simulink library "WBToolbox2Library_repository"  (R2017a)
settings: Solver=ode45  StartTime=0.0  StopTime=10.0  RelTol=1e-3  EnableMultiTasking=on
undefined symbols (not defined in the file): WBT_modelName, WBT_robotName, WBT_wbiFilename, WBT_wbiList
libraries: simulink x1
(part 2 of 2)

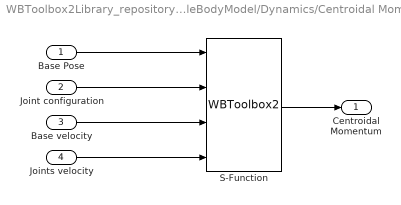
== system WBToolbox2Library_repository/wholeBodyModel/Dynamics/Centroidal Momentum ==
  Base Pose : Inport
  Joint configuration : Inport  Port=2
  Base velocity : Inport  Port=3
  Joints velocity : Inport  Port=4
  S-Function : S-Function  FunctionName=WBToolbox2  Parameters='CentroidalMomentum',robotName,localName,wbiFile,wbiList  SFunctionDeploymentMode=off  EnableBusSupport=off
  Centroidal Momentum : Outport
  wires:
  S-Function/1 -> Centroidal Momentum/1
  Base Pose/1 -> S-Function/1
  Joint configuration/1 -> S-Function/2
  Base velocity/1 -> S-Function/3
  Joints velocity/1 -> S-Function/4

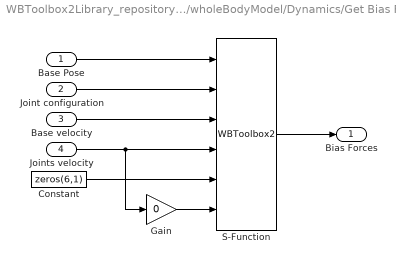
== system WBToolbox2Library_repository/wholeBodyModel/Dynamics/Get Bias Forces ==
  Base Pose : Inport
  Joint configuration : Inport  Port=2
  Base velocity : Inport  Port=3
  Joints velocity : Inport  Port=4
  Constant : Constant  Value=zeros(6,1)
  Gain : Gain  Gain=0
  S-Function : S-Function  FunctionName=WBToolbox2  Parameters='InverseDynamics',robotName,localName,wbiFile,wbiList,explicitGravity  SFunctionDeploymentMode=off  EnableBusSupport=off
  Bias Forces : Outport
  wires:
  S-Function/1 -> Bias Forces/1
  Base Pose/1 -> S-Function/1
  Joint configuration/1 -> S-Function/2
  Base velocity/1 -> S-Function/3
  Joints velocity/1 -> Gain/1, S-Function/4
  Constant/1 -> S-Function/5
  Gain/1 -> S-Function/6

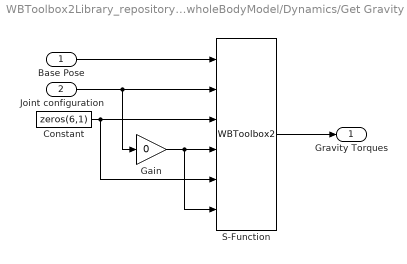
== system WBToolbox2Library_repository/wholeBodyModel/Dynamics/Get Gravity Forces ==
  Base Pose : Inport
  Joint configuration : Inport  Port=2
  Constant : Constant  Value=zeros(6,1)
  Gain : Gain  Gain=0
  S-Function : S-Function  FunctionName=WBToolbox2  Parameters='InverseDynamics',robotName,localName,wbiFile,wbiList,explicitGravity  SFunctionDeploymentMode=off  EnableBusSupport=off
  Gravity Torques : Outport
  wires:
  S-Function/1 -> Gravity Torques/1
  Base Pose/1 -> S-Function/1
  Joint configuration/1 -> Gain/1, S-Function/2
  Constant/1 -> S-Function/5, S-Function/3
  Gain/1 -> S-Function/6, S-Function/4

== system WBToolbox2Library_repository/wholeBodyModel/Dynamics/Mass Matrix ==
  Base Pose : Inport
  Joint configuration : Inport  Port=2
  S-Function : S-Function  FunctionName=WBToolbox2  Parameters='MassMatrix',robotName,localName,wbiFile,wbiList  SFunctionDeploymentMode=off  EnableBusSupport=off
  Mass Matrix : Outport
  wires:
  S-Function/1 -> Mass Matrix/1
  Base Pose/1 -> S-Function/1
  Joint configuration/1 -> S-Function/2

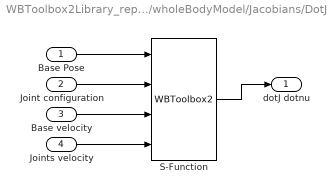
== system WBToolbox2Library_repository/wholeBodyModel/Jacobians/DotJ Nu ==
  Base Pose : Inport
  Joint configuration : Inport  Port=2
  Base velocity : Inport  Port=3
  Joints velocity : Inport  Port=4
  S-Function : S-Function  FunctionName=WBToolbox2  Parameters='DotJNu',robotName,localName,wbiFile,wbiList,frameName  SFunctionDeploymentMode=off  EnableBusSupport=off
  dotJ dotnu : Outport
  wires:
  Joint configuration/1 -> S-Function/2
  Base Pose/1 -> S-Function/1
  S-Function/1 -> dotJ dotnu/1
  Base velocity/1 -> S-Function/3
  Joints velocity/1 -> S-Function/4

== system WBToolbox2Library_repository/wholeBodyModel/Jacobians/Jacobian ==
  Base Pose : Inport
  Joint configuration : Inport  Port=2
  S-Function : S-Function  FunctionName=WBToolbox2  Parameters='Jacobian',robotName,localName,wbiFile,wbiList,frameName  SFunctionDeploymentMode=off  EnableBusSupport=off
  Forward Kinematics : Outport
  wires:
  S-Function/1 -> Forward Kinematics/1
  Base Pose/1 -> S-Function/1
  Joint configuration/1 -> S-Function/2

== system WBToolbox2Library_repository/wholeBodyModel/Kinematics/Forward Kinematics ==
  Base Pose : Inport
  Joint configuration : Inport  Port=2
  S-Function : S-Function  FunctionName=WBToolbox2  Parameters='ForwardKinematics',robotName,localName,wbiFile,wbiList,frameName  SFunctionDeploymentMode=off  EnableBusSupport=off
  Forward Kinematics : Outport
  wires:
  S-Function/1 -> Forward Kinematics/1
  Base Pose/1 -> S-Function/1
  Joint configuration/1 -> S-Function/2

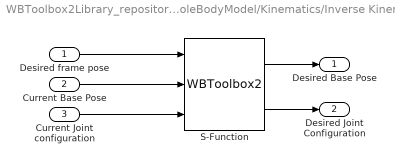
== system WBToolbox2Library_repository/wholeBodyModel/Kinematics/Inverse Kinematics ==
  Desired frame pose : Inport
  Current Base Pose : Inport  Port=2
  Current Joint configuration : Inport  Port=3
  S-Function : S-Function  FunctionName=WBToolbox2  Parameters='InverseKinematics',robotName,localName,wbiFile,wbiList,baseFrame, endEffFrame,optOption  SFunctionDeploymentMode=off  EnableBusSupport=off
  Desired Base Pose : Outport
  Desired Joint Configuration : Outport  Port=2
  wires:
  S-Function/1 -> Desired Base Pose/1
  Current Base Pose/1 -> S-Function/2
  Current Joint configuration/1 -> S-Function/3
  Desired frame pose/1 -> S-Function/1
  S-Function/2 -> Desired Joint Configuration/1

== system WBToolbox2Library_repository/wholeBodyModel/Kinematics/Remote Inverse Kinematics ==
  Desired frame pose : Inport
  Current Joint configuration : Inport  Port=2
  S-Function : S-Function  FunctionName=WBToolbox2  Parameters='RemoteInverseKinematics',solverName, dofs, optOption  SFunctionDeploymentMode=off  EnableBusSupport=off
  Desired Joint Configuration : Outport
  wires:
  S-Function/1 -> Desired Joint Configuration/1
  Desired frame pose/1 -> S-Function/1
  Current Joint configuration/1 -> S-Function/2

== matlab function WBToolbox2Library_repository/Utilities/holder /MATLAB Function ==
  data: s input; s0 output; unused input
function s0 = fcn(s, ~)
persistent state
%#codegen

if isempty(state)
    state = s;
end

s0 = state;

== matlab function WBToolbox2Library_repository/Utilities/DampPinv/Damped Pseudo Inverse ==
  data: mat input; DPinv output; sigma input
function DPinv  = fcn(mat,sigma)
% Economody size svd of mat
[U,S,V] = svd(mat,'econ');
% Damped version of S with sigma
S(S>sigma)=S(S>sigma)./((S(S>sigma)).^2+sigma^2);
% Damped pseudoinverse
DPinv = V*pinv(S)*U';

== matlab function WBToolbox2Library_repository/Utilities/TruncPinv/Truncated PseudoInverse ==
  data: mat input; TPinv output; tol input
function TPinv  = fcn(mat,tol)
%#codegen
[U,S,V] = svd(mat,'econ');
% Setting to zero value
% Setting to 1/S(i,i) singular values greater than tol
 S(S>tol)=1./S(S>tol);
 TPinv = V*pinv(S)*U';
